simulink model "C172pAeroCoefficientsModel"  (R2026a)
settings: configuration reference "standardSILConfiguraitonParams" (kept outside this file)
settings Model: Creator=Edison Altamirano  LastModifiedBy=Edison Altamirano
settings ConfigSetRef: SourceName=standardSILConfiguraitonParams  SourceLocation=Base Workspace

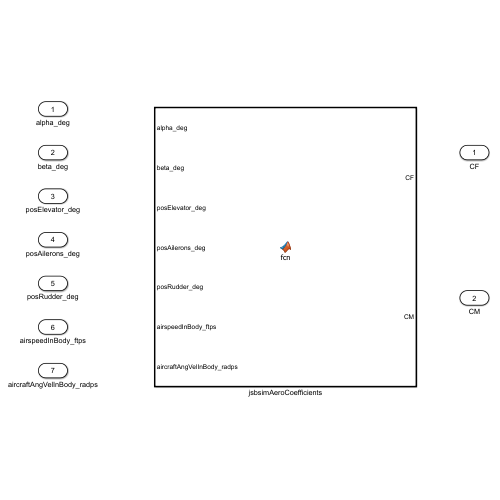
[thumbnail: Simulink's stored preview of the top-level diagram]
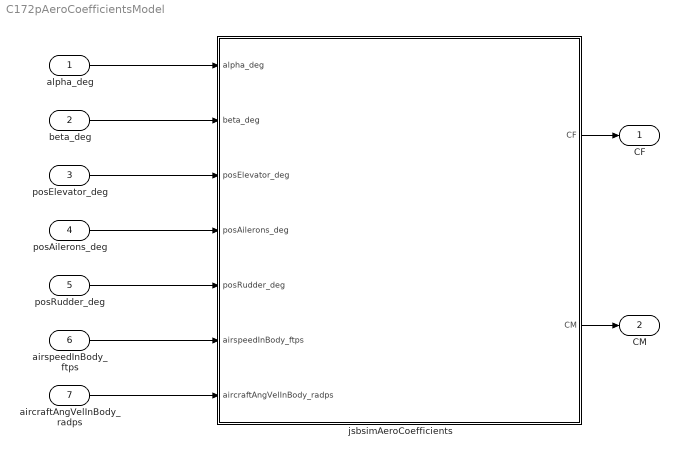
== system C172pAeroCoefficientsModel ==
  alpha_deg : Inport
  beta_deg : Inport  Port=2
  posElevator_deg : Inport  Port=3
  posAilerons_deg : Inport  Port=4
  posRudder_deg : Inport  Port=5
  airspeedInBody_ftps : Inport  Port=6  PortDimensions=3
  aircraftAngVelInBody_radps : Inport  Port=7  PortDimensions=3
  jsbsimAeroCoefficients : MATLAB Function  TreatAsAtomicUnit=on
  CF : Outport
  CM : Outport  Port=2
  wires:
  aircraftAngVelInBody_radps/1 -> jsbsimAeroCoefficients/7(aircraftAngVelInBody_radps)
  posRudder_deg/1 -> jsbsimAeroCoefficients/5(posRudder_deg)
  posElevator_deg/1 -> jsbsimAeroCoefficients/3(posElevator_deg)
  alpha_deg/1 -> jsbsimAeroCoefficients/1(alpha_deg)
  airspeedInBody_ftps/1 -> jsbsimAeroCoefficients/6(airspeedInBody_ftps)
  posAilerons_deg/1 -> jsbsimAeroCoefficients/4(posAilerons_deg)
  beta_deg/1 -> jsbsimAeroCoefficients/2(beta_deg)
  jsbsimAeroCoefficients/1(CF) -> CF/1
  jsbsimAeroCoefficients/2(CM) -> CM/1

== matlab function C172pAeroCoefficientsModel/jsbsimAeroCoefficients ==
  data: alpha_deg input; CF output; beta_deg input; posElevator_deg input; posAilerons_deg input; posRudder_deg input; airspeedInBody_ftps input; aircraftAngVelInBody_radps input; CM output
function [CF, CM] = jsbsimAeroCoefficients(alpha_deg, beta_deg, posElevator_deg, posAilerons_deg, posRudder_deg, airspeedInBody_ftps, aircraftAngVelInBody_radps)
%#codegen
% Cessna 172P aero coefficient buildup, ported from jsbsim/aircraft/c172p/c172p.xml.
% See vehicle/c172p/data/aeroDataC172p.m for full sourcing/derivation of every constant and
% PLAN_INCORPORACION_AERONAVES_JSBSIM_SITL.md for documented fidelity gaps (no ground effect,
% no flap channel, no alpha-rate terms, no stall hysteresis -- pre-stall curve only).
% All constants inlined as local values, not read from a struct-returning params function --
% see optimAeroPX4SIL/CLAUDE.md section 3 on why MATLAB Function blocks in this MATLAB release
% cannot reliably compile a call to a large-nested-struct-returning function.

% c172p.xml <metrics>, converted to SI
bRef_m = 10.9118;
cRef_m = 1.4935;

% DRAG axis
CD0 = 0.027;
CDde_coeff = 0.06;
CDbeta_coeff = 0.17;
CDwbh_alpha_bkpts_rad = [-0.0873 -0.0698 -0.0524 -0.0349 -0.0175 0.0000 0.0175 0.0349 0.0524 0.0698 0.0873 0.1047 0.1222 0.1396 0.1571 0.1745 0.1920 0.2094 0.2269 0.2443 0.2618 0.2793 0.2967 0.3142 0.3316 0.3491];
CDwbh_data = [0.0041 0.0013 0.0001 0.0003 0.0020 0.0052 0.0099 0.0162 0.0240 0.0334 0.0442 0.0566 0.0706 0.0860 0.0962 0.1069 0.1180 0.1298 0.1424 0.1565 0.1727 0.1782 0.1716 0.1618 0.1475 0.1097];

% SIDE axis
CYbeta_coeff = -0.1370 / 0.3490;
CYdr_coeff = 0.187;
CYp_alpha_bkpts_rad = [0.0000 0.0940];
CYp_data = [-0.0750 -0.1450];
CYr_alpha_bkpts_rad = [0.0000 0.0940];
CYr_data = [0.2140 0.2670];

% LIFT axis (CLwbh_data already includes the CL0 intercept -- no separate additive term)
CLwbh_alpha_bkpts_rad = [-0.0900 0.0000 0.0900 0.1000 0.1200 0.1400 0.1600 0.1700 0.1900 0.2100 0.2400 0.2600 0.2800 0.3000 0.3200 0.3400 0.3600];
CLwbh_data = [-0.2200 0.2500 0.7300 0.8300 0.9200 1.0200 1.0800 1.1300 1.1900 1.2500 1.3500 1.4400 1.4700 1.4300 1.3800 1.3000 1.1500];
CLde_coeff = 0.43;
CLq_coeff = 3.9;

% ROLL axis
ClBeta_coeff = -0.0322 / 0.3490;
Clp_coeff = -0.484;
Clr_alpha_bkpts_rad = [0.0000 0.0940];
Clr_data = [0.0798 0.1869];
ClDa_coeff = 0.229;
Cldr_coeff = 0.0147;

% PITCH axis
Cmo_coeff = 0.10;
Cmalpha_coeff = -1.8;
Cmq_coeff = -12.4;
Cmde_coeff = -1.122;

% YAW axis
Cnbeta_coeff = 0.0205 / 0.3490;
Cnp_coeff = -0.0278;
Cnr_coeff = -0.0937;
Cnda_coeff = -0.0053;
Cndr_coeff = -0.0430;

alpha_rad = deg2rad(alpha_deg);
beta_rad = deg2rad(beta_deg);
elevator_rad = deg2rad(posElevator_deg);
aileron_rad = deg2rad(posAilerons_deg);
rudder_rad = deg2rad(posRudder_deg);

V_mps = norm(airspeedInBody_ftps) * 0.3048;
VforRates_mps = max(V_mps, 1.0);
pRate_radps = aircraftAngVelInBody_radps(1);
qRate_radps = aircraftAngVelInBody_radps(2);
rRate_radps = aircraftAngVelInBody_radps(3);
bi2vel = bRef_m / (2 * VforRates_mps);
ci2vel = cRef_m / (2 * VforRates_mps);

CDwbh = interp1(CDwbh_alpha_bkpts_rad, CDwbh_data, alpha_rad, 'linear', 'extrap');
CLwbh = interp1(CLwbh_alpha_bkpts_rad, CLwbh_data, alpha_rad, 'linear', 'extrap');
CYp_v = interp1(CYp_alpha_bkpts_rad, CYp_data, abs(alpha_rad), 'linear', 'extrap');
CYr_v = interp1(CYr_alpha_bkpts_rad, CYr_data, abs(alpha_rad), 'linear', 'extrap');
Clr_v = interp1(Clr_alpha_bkpts_rad, Clr_data, abs(alpha_rad), 'linear', 'extrap');

CD = CD0 + CDwbh + CDde_coeff * abs(elevator_rad) + CDbeta_coeff * abs(beta_rad);
CY = CYbeta_coeff * beta_rad + CYdr_coeff * rudder_rad + CYp_v * bi2vel * pRate_radps + CYr_v * bi2vel * rRate_radps;
CL = CLwbh + CLde_coeff * elevator_rad + CLq_coeff * ci2vel * qRate_radps;

rollMomentCoefficient_nd = ClBeta_coeff * beta_rad + Clp_coeff * bi2vel * pRate_radps + Clr_v * bi2vel * rRate_radps + ClDa_coeff * aileron_rad + Cldr_coeff * rudder_rad;
pitchMomentCoefficient_nd = Cmo_coeff + Cmalpha_coeff * alpha_rad + Cmq_coeff * ci2vel * qRate_radps + Cmde_coeff * elevator_rad;
yawMomentCoefficient_nd = Cnbeta_coeff * beta_rad + Cnp_coeff * bi2vel * pRate_radps + Cnr_coeff * bi2vel * rRate_radps + Cnda_coeff * aileron_rad + Cndr_coeff * rudder_rad;

% Wind-axes (CL,CD) -> body-axes (CX,CZ); CY needs no rotation at this fidelity level.
CXTotal = -CD * cos(alpha_rad) + CL * sin(alpha_rad);
CZTotal = -CD * sin(alpha_rad) - CL * cos(alpha_rad);

CF = [CXTotal; CY; CZTotal];
CM = [rollMomentCoefficient_nd; pitchMomentCoefficient_nd; yawMomentCoefficient_nd];
end
